simulink model "LinearisierteDGL01"  (Simulink 7.1)
settings: Solver=ode15s  StartTime=0.0  StopTime=1.0  RelTol=1e-4
settings Model: Creator=Meisel  LastModifiedBy=Meisel

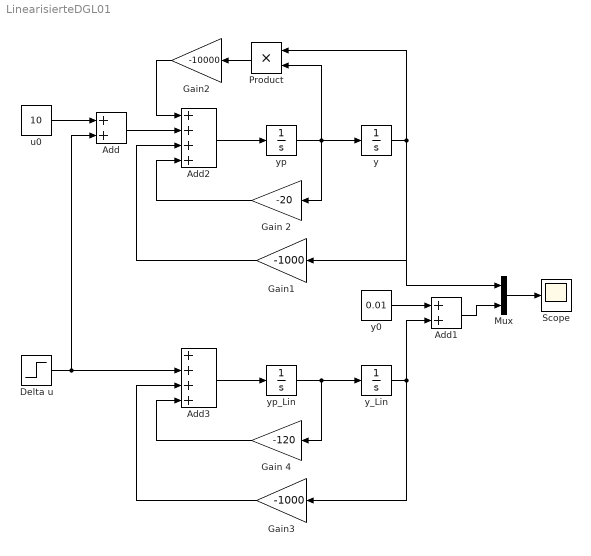
== system LinearisierteDGL01 ==
  Add : Sum  OutDataType=sfix(16)  OutScaling=2^-10
  Add1 : Sum  OutDataType=sfix(16)  OutScaling=2^-10
  Add2 : Sum  Inputs=++++  OutDataType=sfix(16)  OutScaling=2^-10
  Add3 : Sum  Inputs=++++  OutDataType=sfix(16)  OutScaling=2^-10
  Delta u : Step  Time=0.001  After=5  SampleTime=0
  Gain 2 : Gain  Orientation=left  Gain=-20  ParameterDataType=sfix(16)  ParameterScaling=2^0  OutDataType=sfix(16)  OutScaling=2^0
  Gain 4 : Gain  Orientation=left  Gain=-120  ParameterDataType=sfix(16)  ParameterScaling=2^0  OutDataType=sfix(16)  OutScaling=2^0
  Gain1 : Gain  Orientation=left  Gain=-1000  ParameterDataType=sfix(16)  ParameterScaling=2^0  OutDataType=sfix(16)  OutScaling=2^0
  Gain2 : Gain  Orientation=left  Gain=-10000  ParameterDataType=sfix(16)  ParameterScaling=2^0  OutDataType=sfix(16)  OutScaling=2^0
  Gain3 : Gain  Orientation=left  Gain=-1000  ParameterDataType=sfix(16)  ParameterScaling=2^0  OutDataType=sfix(16)  OutScaling=2^0
  Mux : Mux  Inputs=2
  Product : Product  Orientation=left  OutDataType=sfix(16)  OutScaling=2^0  RndMeth=Zero
  Scope : Scope
      settings: TimeRange=1  YMin=0.01  YMax=0.015
  u0 : Constant  Value=10  OutDataType=sfix(16)  OutScaling=2^0
  y : Integrator  InitialCondition=0.01
  y0 : Constant  Value=0.01  OutDataType=sfix(16)  OutScaling=2^0
  y_Lin : Integrator
  yp : Integrator
  yp_Lin : Integrator
  wires:
  yp/1 -> y/1, Gain 2/1, Product/2
  y/1 -> Gain1/1, Product/1, Mux/1
  Gain 2/1 -> Add2/4
  Gain1/1 -> Add2/3
  Gain2/1 -> Add2/1
  Product/1 -> Gain2/1
  Add2/1 -> yp/1
  Add/1 -> Add2/2
  Delta u/1 -> Add/2, Add3/2
  u0/1 -> Add/1
  yp_Lin/1 -> y_Lin/1, Gain 4/1
  y_Lin/1 -> Gain3/1, Add1/2
  Gain 4/1 -> Add3/4
  Gain3/1 -> Add3/3
  Add3/1 -> yp_Lin/1
  Mux/1 -> Scope/1
  y0/1 -> Add1/1
  Add1/1 -> Mux/2
